simulink model "cell_72"  (R2017a)
settings: Solver=VariableStepAuto  StartTime=0.0  StopTime=10.0  RelTol=1e-3
libraries: elec_lib x72, fl_lib x9, nesl_utility x4, simulink x1
settings Model: Creator=Nikhil Kilari  LastModifiedBy=Nikhil Kilari

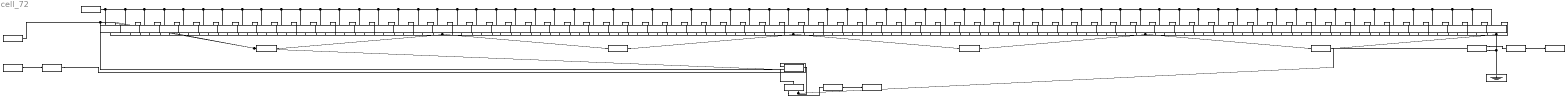
== system cell_72 ==
  Sol1 : elec_lib/Sources/Solar Cell  prm=3  Isc=7.34 A  Voc=0.6 V  Is=1e-6 A  Is2=0 A  Iph=7.34 A  Ir0=1000 W/m^2  ec=1.5  N2=2  Rs=0 Ohm  Rp=Inf Ohm  N_series=1  TIPH1=0 1/K  EG=1.11 eV  TXIS1=3  TXIS2=3  TRS1=0  TRP1=0  Tmeas=200 degC  TFIXED=200 degC  thermal_mass=100 J/K  initial_temperature=25 degC
      settings: SourceProductName=Simscape Electronics  SourceProductBaseCode=SN
  Sol{2..71} (70 alike) : elec_lib/Sources/Solar Cell  prm=1  Isc=7.34 A  Voc=0.6 V  Is=1e-6 A  Is2=0 A  Iph=7.34 A  Ir0=1000 W/m^2  ec=1.5  N2=2  Rs=0 Ohm  Rp=Inf Ohm  N_series=1  TIPH1=0 1/K  EG=1.11 eV  TXIS1=3  TXIS2=3  TRS1=0  TRP1=0  Tmeas=25 degC  TFIXED=25 degC  thermal_mass=100 J/K  initial_temperature=25 degC
      settings: SourceProductName=Simscape Electronics  SourceProductBaseCode=SN
  Sol72 : elec_lib/Sources/Solar Cell  prm=1  Isc=7.34 A  Voc=0.6 V  Is=1e-6 A  Is2=0 A  Iph=7.34 A  Ir0=1000 W/m^2  ec=1.5  N2=2  Rs=0 Ohm  Rp=10000 Ohm  N_series=1  TIPH1=0 1/K  EG=1.11 eV  TXIS1=3  TXIS2=3  TRS1=0  TRP1=0  Tmeas=200 degC  TFIXED=200 degC  thermal_mass=100 J/K  initial_temperature=25 degC
      settings: SourceProductName=Simscape Electronics  SourceProductBaseCode=SN
  bpd{1..4} (4 alike) : fl_lib/Electrical/Electrical Elements/Diode  Vf=0.6 V  Ron=0.3 Ohm  Goff=1e-8 1/Ohm  i_specify=off  i_priority=None  i=0 A  i_nominal_specify=off  i_nominal_unit=A  i_nominal_value=1  v_specify=off  v_priority=None  v=0 V  v_nominal_specify=off  v_nominal_unit=V  v_nominal_value=1
  cs : fl_lib/Electrical/Electrical Sensors/Current Sensor
  csconv : nesl_utility/PS-Simulink Converter  PhysicalDomain=network_engine_domain  SubClassName=ps_output  LeftPortType=input  RightPortType=output  PseudoPeriodic=off  Frequencies=[]  Unit=1  AffineConversion=off
  cswspc : ToWorkspace  VariableName=Current  SampleTime=-1
  elecref : fl_lib/Electrical/Electrical Elements/Electrical Reference
  irr : fl_lib/Physical Signals/Sources/PS Constant  constant=1000
  ramp : simulink/Sources/Ramp  slope=1000  start=0  X0=0
  rampconv : nesl_utility/Simulink-PS Converter  PhysicalDomain=network_engine_domain  SubClassName=ps_input  LeftPortType=input  RightPortType=output  PseudoPeriodic=off  Frequencies=[]  NoiseDistribution=none  NoiseParameters=[]  Unit=1  AffineConversion=off  FilteringAndDerivatives=provide  SimscapeFilterOrder=1  InputFilterTimeConstant=0.001  UdotUserProvided=0
  solverconfig : nesl_utility/Solver Configuration  PhysicalDomain=network_engine_domain  SubClassName=solver  LeftPortType=input  RightPortType=generic  Accelerate=off  Tones=[]  Harmonics=[]  SimulateNoise=off  Profile=off  UseLocalSampling=off  EnableSwitchedLinearOptims=on  FrequencyDomain=off  UseCCode=off  RelTol=0.001  AbsTol=1e-06  MinStep=1e-09  ToWorkspace=off  RevertToSquareIcSolve=off  NumHomotopyIterations=100  PhasorMode=off  PhasorModeNumHarmonics=1  OverrideAbsTol=off  DoDC=off  ResidualTolerance=1e-09  UseLocalSolver=on  LocalSolverChoice=NE_BACKWARD_EULER_ADVANCER  LocalSolverSampleTime=0.001  DoFixedCost=on  MaxNonlinIter=3  MaxModeIter=2  LinearAlgebra=Sparse  DelaysMemoryBudget=1024  AutomaticFiltering=on  FilteringTimeConstant=0.001
  var_res : fl_lib/Electrical/Electrical Elements/Variable Resistor  Rmin=0 Ohm  i_specify=off  i_priority=None  i=0 A  i_nominal_specify=off  i_nominal_unit=A  i_nominal_value=1  v_specify=off  v_priority=None  v=0 V  v_nominal_specify=off  v_nominal_unit=V  v_nominal_value=1
  vs : fl_lib/Electrical/Electrical Sensors/Voltage Sensor
  vsconv : nesl_utility/PS-Simulink Converter  PhysicalDomain=network_engine_domain  SubClassName=ps_output  LeftPortType=input  RightPortType=output  PseudoPeriodic=off  Frequencies=[]  Unit=1  AffineConversion=off
  vswspc : ToWorkspace  VariableName=Voltage  SampleTime=-1
  wires:
  ramp/1 -> rampconv/1
  vsconv/1 -> vswspc/1
  csconv/1 -> cswspc/1
  connections:
  Sol1/LConn1 -- irr/RConn1 -- Sol71/LConn1 -- Sol72/LConn1 -- Sol70/LConn1 -- Sol69/LConn1 -- Sol68/LConn1 -- Sol67/LConn1 -- Sol66/LConn1 -- Sol65/LConn1 -- Sol64/LConn1 -- Sol63/LConn1 -- Sol62/LConn1 -- Sol61/LConn1 -- Sol60/LConn1 -- Sol59/LConn1 -- Sol58/LConn1 -- Sol57/LConn1 -- Sol56/LConn1 -- Sol55/LConn1 -- Sol54/LConn1 -- Sol53/LConn1 -- Sol52/LConn1 -- Sol51/LConn1 -- Sol50/LConn1 -- Sol49/LConn1 -- Sol48/LConn1 -- Sol47/LConn1 -- Sol46/LConn1 -- Sol45/LConn1 -- Sol44/LConn1 -- Sol43/LConn1 -- Sol42/LConn1 -- Sol41/LConn1 -- Sol40/LConn1 -- Sol39/LConn1 -- Sol38/LConn1 -- Sol37/LConn1 -- Sol36/LConn1 -- Sol35/LConn1 -- Sol34/LConn1 -- Sol33/LConn1 -- Sol32/LConn1 -- Sol31/LConn1 -- Sol30/LConn1 -- Sol29/LConn1 -- Sol28/LConn1 -- Sol27/LConn1 -- Sol26/LConn1 -- Sol25/LConn1 -- Sol24/LConn1 -- Sol23/LConn1 -- Sol22/LConn1 -- Sol21/LConn1 -- Sol20/LConn1 -- Sol19/LConn1 -- Sol18/LConn1 -- Sol17/LConn1 -- Sol16/LConn1 -- Sol15/LConn1 -- Sol14/LConn1 -- Sol13/LConn1 -- Sol12/LConn1 -- Sol11/LConn1 -- Sol10/LConn1 -- Sol9/LConn1 -- Sol8/LConn1 -- Sol7/LConn1 -- Sol6/LConn1 -- Sol5/LConn1 -- Sol4/LConn1 -- Sol3/LConn1 -- Sol2/LConn1
  Sol2/LConn2 -- Sol1/RConn1
  Sol3/LConn2 -- Sol2/RConn1
  Sol4/LConn2 -- Sol3/RConn1
  Sol5/LConn2 -- Sol4/RConn1
  Sol6/LConn2 -- Sol5/RConn1
  Sol7/LConn2 -- Sol6/RConn1
  Sol8/LConn2 -- Sol7/RConn1
  Sol9/LConn2 -- Sol8/RConn1
  Sol10/LConn2 -- Sol9/RConn1
  Sol11/LConn2 -- Sol10/RConn1
  Sol12/LConn2 -- Sol11/RConn1
  Sol13/LConn2 -- Sol12/RConn1
  Sol14/LConn2 -- Sol13/RConn1
  Sol15/LConn2 -- Sol14/RConn1
  Sol16/LConn2 -- Sol15/RConn1
  Sol17/LConn2 -- Sol16/RConn1
  Sol18/LConn2 -- Sol17/RConn1
  Sol18/RConn1 -- Sol19/LConn2 -- bpd1/LConn1 -- bpd2/RConn1
  Sol20/LConn2 -- Sol19/RConn1
  Sol21/LConn2 -- Sol20/RConn1
  Sol22/LConn2 -- Sol21/RConn1
  Sol23/LConn2 -- Sol22/RConn1
  Sol24/LConn2 -- Sol23/RConn1
  Sol25/LConn2 -- Sol24/RConn1
  Sol26/LConn2 -- Sol25/RConn1
  Sol27/LConn2 -- Sol26/RConn1
  Sol28/LConn2 -- Sol27/RConn1
  Sol29/LConn2 -- Sol28/RConn1
  Sol30/LConn2 -- Sol29/RConn1
  Sol31/LConn2 -- Sol30/RConn1
  Sol32/LConn2 -- Sol31/RConn1
  Sol33/LConn2 -- Sol32/RConn1
  Sol34/LConn2 -- Sol33/RConn1
  Sol35/LConn2 -- Sol34/RConn1
  Sol36/LConn2 -- Sol35/RConn1
  Sol36/RConn1 -- Sol37/LConn2 -- bpd2/LConn1 -- bpd3/RConn1
  Sol38/LConn2 -- Sol37/RConn1
  Sol39/LConn2 -- Sol38/RConn1
  Sol40/LConn2 -- Sol39/RConn1
  Sol41/LConn2 -- Sol40/RConn1
  Sol42/LConn2 -- Sol41/RConn1
  Sol43/LConn2 -- Sol42/RConn1
  Sol44/LConn2 -- Sol43/RConn1
  Sol45/LConn2 -- Sol44/RConn1
  Sol46/LConn2 -- Sol45/RConn1
  Sol47/LConn2 -- Sol46/RConn1
  Sol48/LConn2 -- Sol47/RConn1
  Sol49/LConn2 -- Sol48/RConn1
  Sol50/LConn2 -- Sol49/RConn1
  Sol51/LConn2 -- Sol50/RConn1
  Sol52/LConn2 -- Sol51/RConn1
  Sol53/LConn2 -- Sol52/RConn1
  Sol54/LConn2 -- Sol53/RConn1
  Sol54/RConn1 -- Sol55/LConn2 -- bpd3/LConn1 -- bpd4/RConn1
  Sol56/LConn2 -- Sol55/RConn1
  Sol57/LConn2 -- Sol56/RConn1
  Sol58/LConn2 -- Sol57/RConn1
  Sol59/LConn2 -- Sol58/RConn1
  Sol60/LConn2 -- Sol59/RConn1
  Sol61/LConn2 -- Sol60/RConn1
  Sol62/LConn2 -- Sol61/RConn1
  Sol63/LConn2 -- Sol62/RConn1
  Sol64/LConn2 -- Sol63/RConn1
  Sol65/LConn2 -- Sol64/RConn1
  Sol66/LConn2 -- Sol65/RConn1
  Sol67/LConn2 -- Sol66/RConn1
  Sol68/LConn2 -- Sol67/RConn1
  Sol69/LConn2 -- Sol68/RConn1
  Sol70/LConn2 -- Sol69/RConn1
  Sol71/LConn2 -- Sol70/RConn1
  Sol72/LConn2 -- Sol71/RConn1
  Sol1/LConn2 -- solverconfig/RConn1 -- var_res/LConn2 -- bpd1/RConn1 -- vs/LConn1
  bpd4/LConn1 -- cs/RConn2 -- elecref/LConn1 -- Sol72/RConn1
  rampconv/RConn1 -- var_res/LConn1
  vs/RConn2 -- var_res/RConn1 -- cs/LConn1
  vs/RConn1 -- vsconv/LConn1
  cs/RConn1 -- csconv/LConn1
